simulink model "PID_FUQROS_2015"  (R2015b)
settings: Solver=VariableStepAuto  StartTime=0.0  StopTime=80  RelTol=1e-3
values from neighbouring files (symbols this model uses):
  ki = 0    [path_follower_main.m]
  kp = 1    [path_follower_main.m]
  kv = .05    (= 0.05)    [path_follower_main.m]
  L = 4.5    [controller_test.m]    (also in path_follower_main.m)
  theta0 = -pi    (= -3.14159265359)    [controller_test.m]    (also in path_follower_main.m = 0.523598775598)
  x0 = 10    [controller_test.m]    (also in path_follower_main.m = 0)
  y0 = 10    [controller_test.m]    (also in path_follower_main.m = 0)
libraries: simulink x2
settings Model: Creator=Mitch  LastModifiedBy=gasoto

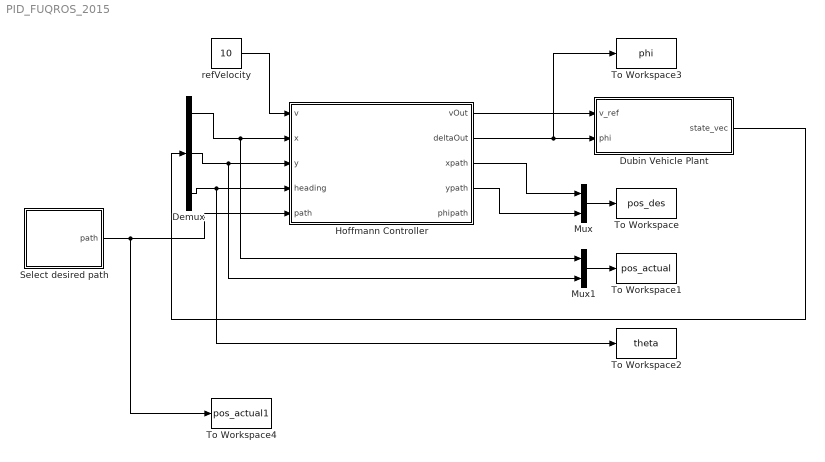
== system PID_FUQROS_2015 ==
  Demux : Demux  Outputs=3
  Dubin Vehicle Plant : Subsystem
  Hoffmann Controller : Subsystem
  Mux : Mux  Inputs=2
  Mux1 : Mux  Inputs=2
  Select desired path : Subsystem
  To Workspace : ToWorkspace  VariableName=pos_des  SampleTime=-1
      settings: Save2DSignal=2-D array (concatenate along first dimension)
  To Workspace1 : ToWorkspace  VariableName=pos_actual  SampleTime=-1
      settings: Save2DSignal=2-D array (concatenate along first dimension)
  To Workspace2 : ToWorkspace  VariableName=theta  SaveFormat=Structure With Time  SampleTime=-1
      settings: Save2DSignal=2-D array (concatenate along first dimension)
  To Workspace3 : ToWorkspace  VariableName=phi  SaveFormat=Structure With Time  SampleTime=-1
      settings: Save2DSignal=2-D array (concatenate along first dimension)
  To Workspace4 : ToWorkspace  VariableName=pos_actual1  SaveFormat=Structure  SampleTime=-1
      settings: Save2DSignal=2-D array (concatenate along first dimension)
  refVelocity : Constant  Value=10
  wires:
  Hoffmann Controller/2(deltaOut) -> To Workspace3/1, Dubin Vehicle Plant/2(phi)
  Dubin Vehicle Plant/1(state_vec) -> Demux/1
  Demux/1 -> Mux1/1, Hoffmann Controller/2(x)
  Demux/2 -> Mux1/2, Hoffmann Controller/3(y)
  Demux/3 -> To Workspace2/1, Hoffmann Controller/4(heading)
  refVelocity/1 -> Hoffmann Controller/1(v)
  Hoffmann Controller/1(vOut) -> Dubin Vehicle Plant/1(v_ref)
  Hoffmann Controller/3(xpath) -> Mux/1
  Hoffmann Controller/4(ypath) -> Mux/2
  Mux1/1 -> To Workspace1/1
  Mux/1 -> To Workspace/1
  Select desired path/1(path) -> To Workspace4/1, Hoffmann Controller/5(path)

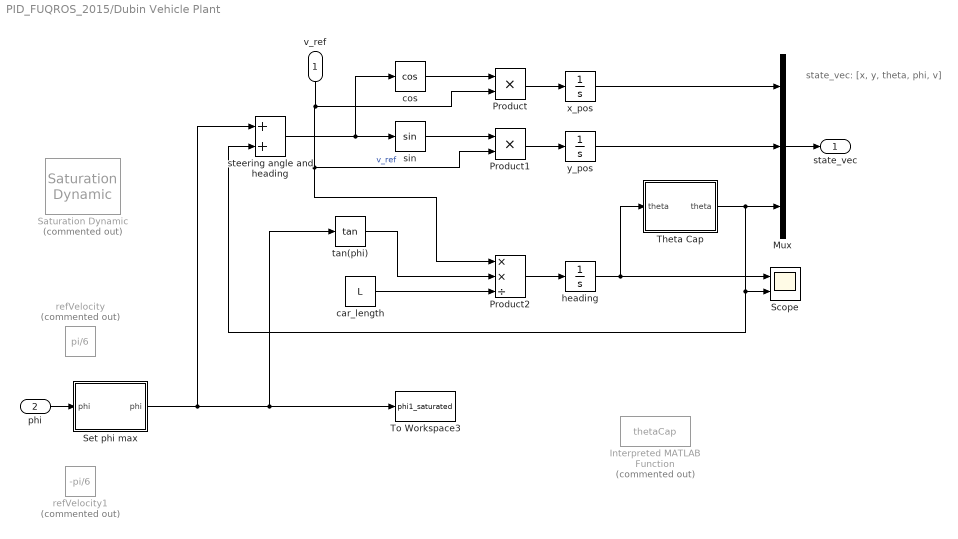
== system PID_FUQROS_2015/Dubin Vehicle Plant ==
  note: state_vec:
      | [x, y, theta, phi, v]
  v_ref : Inport
  phi : Inport  Port=2
  Interpreted MATLAB Function : MATLABFcn  Commented=on  MATLABFcn=thetaCap
  Mux : Mux  Inputs=3
  Product : Product
  Product1 : Product
  Product2 : Product  Inputs=**/
  Saturation Dynamic : simulink/Discontinuities/Saturation Dynamic  Commented=on  OutMin=[]  OutMax=[]  OutDataTypeStr=Inherit: Same as second input  OutDataType=fixdt(1, 16)  OutScaling=2^-10  DoSatur=off
  Scope : Scope  NumInputPorts=2
  Set phi max : MATLAB Function  TreatAsAtomicUnit=on
      settings: PermitHierarchicalResolution=ParametersOnly
  Theta Cap : MATLAB Function  TreatAsAtomicUnit=on
      settings: PermitHierarchicalResolution=ParametersOnly
  To Workspace3 : ToWorkspace  VariableName=phi1_saturated  SaveFormat=Structure With Time  SampleTime=-1
      settings: Save2DSignal=2-D array (concatenate along first dimension)
  car_length : Constant  Value=L
  cos : Trigonometry  Operator=cos
  heading : Integrator  InitialCondition=theta0
  refVelocity : Constant  Commented=on  Value=pi/6
  refVelocity1 : Constant  Commented=on  Value=-pi/6
  sin : Trigonometry
  steering angle and heading : Sum
  tan(phi) : Trigonometry  Operator=tan
  x_pos : Integrator  InitialCondition=x0
  y_pos : Integrator  InitialCondition=y0
  state_vec : Outport
  wires:
  y_pos/1 -> Mux/2
  x_pos/1 -> Mux/1
  Mux/1 -> state_vec/1
  Product/1 -> x_pos/1
  Product1/1 -> y_pos/1
  Product2/1 -> heading/1
  car_length/1 -> Product2/3
  v_ref/1 -> Product2/1, Product1/2, Product/2  "v_ref"
  steering angle and heading/1 -> cos/1, sin/1
  cos/1 -> Product/1
  sin/1 -> Product1/1
  tan(phi)/1 -> Product2/2
  heading/1 -> Theta Cap/1("theta "), Scope/1
  Theta Cap/1(theta) -> Scope/2, steering angle and heading/2, Mux/3
  phi/1 -> Set phi max/1("phi ")
  Set phi max/1(phi) -> steering angle and heading/1, tan(phi)/1, To Workspace3/1

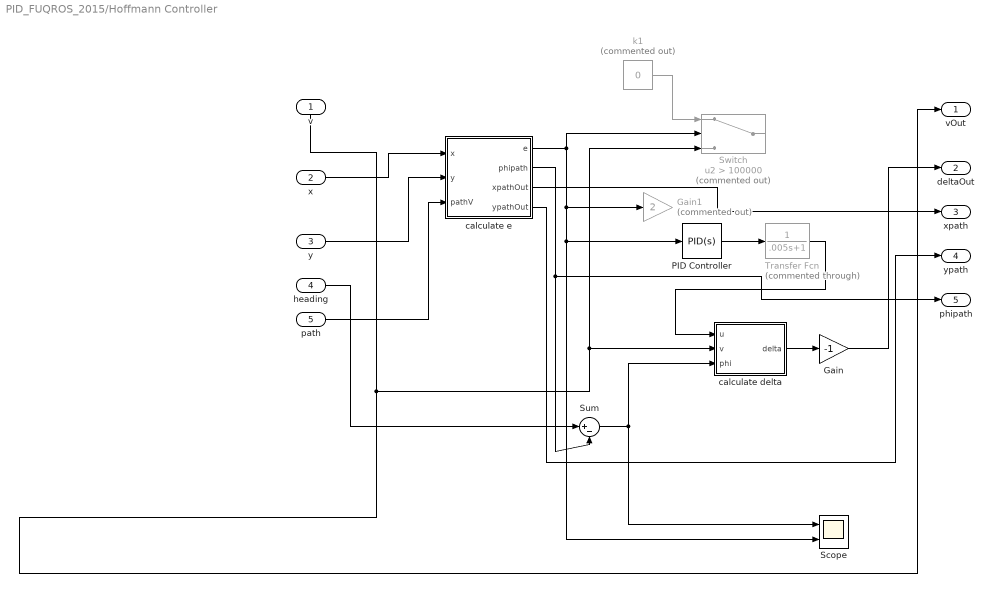
== system PID_FUQROS_2015/Hoffmann Controller ==
  v : Inport
  x : Inport  Port=2
  y : Inport  Port=3
  heading : Inport  Port=4
  path : Inport  Port=5
  Gain : Gain  Gain=-1
  Gain1 : Gain  Commented=on  Gain=2
  PID Controller : simulink/Continuous/PID Controller  Controller=PID  TimeDomain=Continuous-time  SampleTime=-1  IntegratorMethod=Forward Euler  FilterMethod=Forward Euler  Form=Parallel  UseFilter=on  ControllerParametersSource=internal  P=kp  I=ki  D=kv  N=100  InitialConditionSource=internal  InitialConditionForIntegrator=0  InitialConditionForFilter=0  ExternalReset=none  LimitOutput=off  UpperSaturationLimit=inf  LowerSaturationLimit=-inf  LinearizeAsGain=on  AntiWindupMode=none  Kb=1  TrackingMode=off  Kt=1  PParamMin=[]  PParamMax=[]  IParamMin=[]  IParamMax=[]  DParamMin=[]  DParamMax=[]  NParamMin=[]  NParamMax=[]  KbParamMin=[]  KbParamMax=[]  KtParamMin=[]  KtParamMax=[]  POutMin=[]  POutMax=[]  IOutMin=[]  IOutMax=[]  DOutMin=[]  DOutMax=[]  NOutMin=[]  NOutMax=[]  KbOutMin=[]  KbOutMax=[]  KtOutMin=[]  KtOutMax=[]  IntegratorOutMin=[]  IntegratorOutMax=[]  FilterOutMin=[]  FilterOutMax=[]  SumOutMin=[]  SumOutMax=[]  SumI1OutMin=[]  SumI1OutMax=[]  SumI2OutMin=[]  SumI2OutMax=[]  SumI3OutMin=[]  SumI3OutMax=[]  SumDOutMin=[]  SumDOutMax=[]  SaturationOutMin=[]  SaturationOutMax=[]  IntegratorContinuousStateAttributes=''  IntegratorStateMustResolveToSignalObject=off  IntegratorRTWStateStorageClass=Auto  FilterContinuousStateAttributes=''  FilterStateMustResolveToSignalObject=off  FilterRTWStateStorageClass=Auto  DifferentiatorICPrevScaledInput=0  DifferentiatorOutMin=[]  DifferentiatorOutMax=[]
  Scope : Scope  NumInputPorts=2
  Sum : Sum  Inputs=|+-
  Switch : Switch  Commented=on  Criteria=u2 > Threshold  Threshold=100000
  Transfer Fcn : TransferFcn  Commented=through  Denominator=[.005 1]
  calculate delta : MATLAB Function  TreatAsAtomicUnit=on
      settings: PermitHierarchicalResolution=ParametersOnly
  calculate e : MATLAB Function  TreatAsAtomicUnit=on
      settings: PermitHierarchicalResolution=ParametersOnly
  k1 : Constant  Commented=on  Value=0
  vOut : Outport
  deltaOut : Outport  Port=2
  xpath : Outport  Port=3
  ypath : Outport  Port=4
  phipath : Outport  Port=5
  wires:
  v/1 -> vOut/1, Switch/3, calculate delta/2(v)
  path/1 -> calculate e/3(pathV)
  x/1 -> calculate e/1(x)
  y/1 -> calculate e/2(y)
  calculate e/2(phipath) -> phipath/1, Sum/2
  calculate e/1(e) -> Switch/2, Scope/2, PID Controller/1, Gain1/1
  Sum/1 -> Scope/1, calculate delta/3(phi)
  calculate e/3(xpathOut) -> xpath/1
  calculate e/4(ypathOut) -> ypath/1
  k1/1 -> Switch/1
  heading/1 -> Sum/1
  calculate delta/1(delta) -> Gain/1
  Gain/1 -> deltaOut/1
  PID Controller/1 -> Transfer Fcn/1
  Transfer Fcn/1 -> calculate delta/1(u)

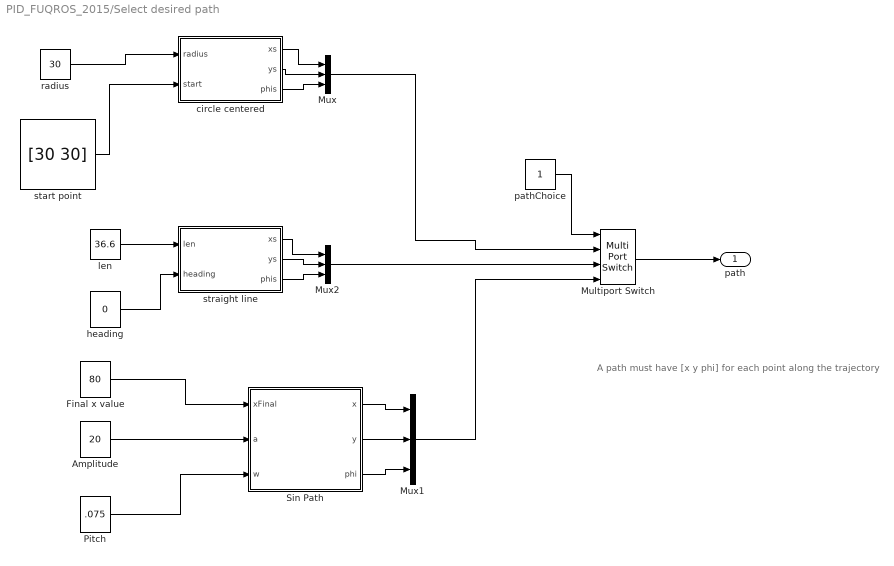
== system PID_FUQROS_2015/Select desired path ==
  note: A path must have [x y phi] for each point along the trajectory
  Amplitude : Constant  Value=20
  "Final x value " : Constant  Value=80
  Multiport Switch : MultiPortSwitch
  Mux : Mux  Inputs=3
  Mux1 : Mux  Inputs=3
  Mux2 : Mux  Inputs=3
  Pitch : Constant  Value=.075
  Sin Path : MATLAB Function  TreatAsAtomicUnit=on
      settings: PermitHierarchicalResolution=ParametersOnly
  circle centered : MATLAB Function  TreatAsAtomicUnit=on
      settings: PermitHierarchicalResolution=ParametersOnly
  heading : Constant  Value=0
  len : Constant  Value=36.6
  "pathChoice " : Constant
  radius : Constant  Value=30
  start point : Constant  Value=[30 30]
  straight line : MATLAB Function  TreatAsAtomicUnit=on
      settings: PermitHierarchicalResolution=ParametersOnly
  path : Outport
  wires:
  radius/1 -> circle centered/1(radius)
  start point/1 -> circle centered/2(start)
  "pathChoice "/1 -> Multiport Switch/1
  circle centered/2(ys) -> Mux/2
  circle centered/1(xs) -> Mux/1
  Multiport Switch/1 -> path/1
  len/1 -> straight line/1(len)
  heading/1 -> straight line/2(heading)
  straight line/1(xs) -> Mux2/1
  straight line/2(ys) -> Mux2/2
  Mux2/1 -> Multiport Switch/3
  Mux/1 -> Multiport Switch/2
  straight line/3(phis) -> Mux2/3
  circle centered/3(phis) -> Mux/3
  Amplitude/1 -> Sin Path/2(a)
  "Final x value "/1 -> Sin Path/1(xFinal)
  Pitch/1 -> Sin Path/3(w)
  Sin Path/1(x) -> Mux1/1
  Sin Path/2(y) -> Mux1/2
  Sin Path/3(phi) -> Mux1/3
  Mux1/1 -> Multiport Switch/4

== matlab function PID_FUQROS_2015/Hoffmann Controller/calculate e ==
  data: e output; x input; y input; pathV input; phipath output; xpathOut output; ypathOut output
function [e,phipath,xpathOut,ypathOut] = fcn(x,y,pathV)
%#codegen
path=reshape(pathV,[],3);
x1 = path(1,1);
y1 = path(1,2);
phi1=path(1,3);
etmp = inf;
e = inf;
index=1;
% find the nearest x,y
for i=1:length(path)
   etmp = sqrt((x-path(i,1))^2+(y-path(i,2))^2);
   if( etmp < e )
       e = etmp;
       index=i;
   end
end

xpathOut=path(index,1);
ypathOut=path(index,2);
phipath=path(index,3);

ex1 = (path(index,1)-x);
ey1 = (path(index,2)-y);
ex2 = cos(phipath);
ey2 = sin(phipath);
sinnnn = ex1*ey2-ey1*ex2;
e = sign(sinnnn)*e;

== matlab function PID_FUQROS_2015/Dubin Vehicle Plant/Theta Cap ==
  data: theta input; theta output
function theta = fcn(theta)
    while abs(theta) > pi
        theta = theta - sign(theta)*2*pi;
    end

== matlab function PID_FUQROS_2015/Hoffmann Controller/calculate delta ==
  data: delta output; u input; v input; phi input
function delta = fcn(u,v,phi)
%#codegen
if( abs(v) < eps )
    v = eps;
end

% if phi is greater than pi (or less than -pi), then 
% we normalize to between [-pi,pi]
if( phi < -pi )
    phi = phi+2*pi;
elseif( phi > pi )
    phi = phi-2*pi;
end

delta = phi + atan2(u,v);

== matlab function PID_FUQROS_2015/Select desired path/circle centered ==
  data: xs output; radius input; start input; ys output; phis output
function [xs,ys,phis] = fcn(radius,start)
%#codegen
angles=linspace(-pi,pi,3000);
r = radius*exp(angles*1j);
xs = real(r)-radius+start(1);
ys = imag(r)+start(2);
phis=(pi/2)+angles;

% % % To visualize the angles, run this code:
% radius=3.6; start=[0 0];
% angles=linspace(-pi,pi,10);
% r = radius*exp(angles*1j);
% xs = real(r)-radius+start(1);
% ys = imag(r)+start(2);
% % since the direction of travel is in the 'x' direction, the 
% % heading (phi) matchines the angle of the circle
% phis=(pi/2)+angles;
% xends=.5*cos(phis);yends=.5*sin(phis);
% figure;plot(xs,ys);hold on; quiver(xs,ys,xends,yends);axis equal;hold off

== matlab function PID_FUQROS_2015/Select desired path/straight line ==
  data: xs output; len input; heading input; ys output; phis output
function [xs,ys,phis] = fcn(len,heading)
%#codegen
r = linspace(0,len,3000);
xs = r*cos(heading);
ys = r*sin(heading);
phis = heading*ones(1,length(r));

== matlab function PID_FUQROS_2015/Select desired path/Sin Path ==
  data: x output; xFinal input; y output; a input; w input; phi output
function [x,y,phi] = getSinPath(xFinal,a,w)

% x = 0:.01:xFinal;
x = linspace(0,xFinal,3000);
y = a*sin(w*x);
slope = cos(x);
phi = atan(slope);
end

== matlab function PID_FUQROS_2015/Dubin Vehicle Plant/Set phi max ==
  data: phi input; phi output
function phi = phiCap(phi)

if phi > pi/6
    phi = pi/6;
elseif phi < -pi/6
    phi = -pi/6;
end
